simulink model "threephasedcac"  (R2016a)
settings: Solver=VariableStepAuto  StartTime=0.0  StopTime=60e-3  RelTol=1e-3
libraries: powerlib x15, powerlib_meascontrol x4
settings Model: Creator=VARUN SINGH  LastModifiedBy=VARUN SINGH

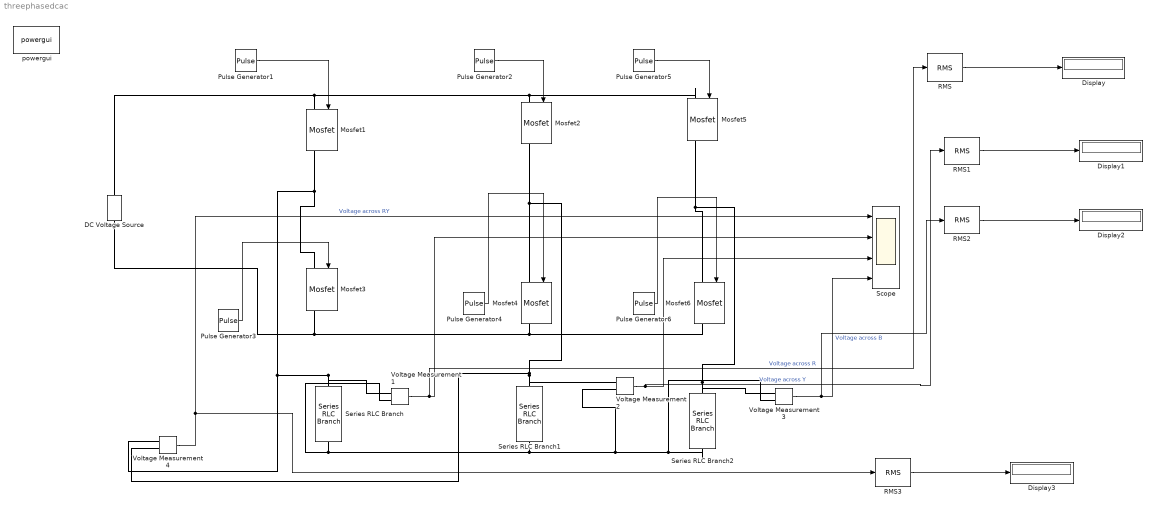
== system threephasedcac ==
  DC Voltage Source : powerlib/Electrical Sources/DC Voltage Source  Amplitude=325  Measurements=None
  Display{,1..3} (4 alike) : Display
  Mosfet{1..6} (6 alike) : powerlib/Power Electronics/Mosfet  Ron=0.1  Lon=0  Rd=0.01  Vfd=0  IC=0  Rs=1e5  Cs=inf  Measurements=on
  Pulse Generator1 : DiscretePulseGenerator  PulseType=Time based  Period=20e-3  PulseWidth=100/3
  Pulse Generator2 : DiscretePulseGenerator  PulseType=Time based  Period=20e-3  PulseWidth=100/3  PhaseDelay=(180/180)*10e-3
  Pulse Generator3 : DiscretePulseGenerator  PulseType=Time based  Period=20e-3  PulseWidth=100/3  PhaseDelay=10e-3
  Pulse Generator4 : DiscretePulseGenerator  PulseType=Time based  Period=20e-3  PulseWidth=100/3  PhaseDelay=(180/180)*10e-3+10e-3
  Pulse Generator5 : DiscretePulseGenerator  PulseType=Time based  Period=20e-3  PulseWidth=100/3  PhaseDelay=(360/180)*10e-3
  Pulse Generator6 : DiscretePulseGenerator  PulseType=Time based  Period=20e-3  PulseWidth=100/3  PhaseDelay=(360/180)*10e-3+10e-3
  RMS{,1..3} (4 alike) : powerlib_meascontrol/Measurements/RMS  TrueRMS=on  Freq=60  RMSInit=120  Ts=0
  Scope : Scope  NumInputPorts=4
  Series RLC Branch : powerlib/Elements/Series RLC Branch  LConnTagsString=__new0  RConnTagsString=__new0  BranchType=R  Resistance=100  Inductance=10e-3  SetiL0=off  InitialCurrent=0  Capacitance=1e-6  Setx0=off  InitialVoltage=0  Measurements=None
  Series RLC Branch1 : powerlib/Elements/Series RLC Branch  LConnTagsString=__new0  RConnTagsString=__new0  BranchType=R  Resistance=100  Inductance=10e-3  SetiL0=off  InitialCurrent=0  Capacitance=1e-6  Setx0=off  InitialVoltage=0  Measurements=None
  Series RLC Branch2 : powerlib/Elements/Series RLC Branch  LConnTagsString=__new0  RConnTagsString=__new0  BranchType=R  Resistance=100  Inductance=10e-3  SetiL0=off  InitialCurrent=0  Capacitance=1e-6  Setx0=off  InitialVoltage=0  Measurements=None
  Voltage Measurement{1..4} (4 alike) : powerlib/Measurements/Voltage Measurement  PhasorSimulation=off  OutputType=Complex  PSBequivalent=0
  powergui : powerlib/powergui  Priority=1  SimulationMode=Continuous  SolverType=Tustin/Backward Euler (TBE)  SampleTime=50e-6  frequency=60  SPID=off  DisableSnubberDevices=off  DisableRonSwitches=off  DisableVfSwitches=off  SwTol=0  DisplayEquations=off  Interpol=off  ExternalGateDelay=off  methode=off  Ts=10  FunctionMessages=off  echomessages=off  HookPort=off  EnableUseOfTLC=off  x0status=blocks  frequencyindice=0  Pbase=100e6  ErrMax=1e-4  Iterations=50  UnitsV=kV  UnitsW=MW  buscounter=0  RestoreLinks=warning  ResistiveCurrentMeasurement=off  Frange=[0:2:500]  Ylog=off  Xlog=on  ShowGrid=off  save=off  variable=ZData  structure=0  ZoomFFT=off  StartTime=0.0  cycles=1  DisplayStyle=1  fundamental=60  FreqAxis=off  MaxFrequency=1000  frequencyindicesteady=1  RmsSteady=1  display=off
  wires:
  Pulse Generator5/1 -> Mosfet5/1
  Pulse Generator6/1 -> Mosfet6/1
  Pulse Generator2/1 -> Mosfet2/1
  Pulse Generator4/1 -> Mosfet4/1
  Pulse Generator1/1 -> Mosfet1/1
  Pulse Generator3/1 -> Mosfet3/1
  Voltage Measurement4/1 -> RMS3/1, Scope/1  "Voltage across RY"
  Voltage Measurement1/1 -> RMS/1, Scope/2  "Voltage across R"
  Voltage Measurement2/1 -> RMS1/1, Scope/3  "Voltage across Y"
  Voltage Measurement3/1 -> RMS2/1, Scope/4  "Voltage across B"
  RMS/1 -> Display/1
  RMS2/1 -> Display2/1
  RMS1/1 -> Display1/1
  RMS3/1 -> Display3/1
  connections:
  Mosfet2/RConn1 -- Voltage Measurement4/LConn2 -- Voltage Measurement2/LConn1 -- Series RLC Branch1/RConn1 -- Mosfet4/LConn1
  Mosfet3/LConn1 -- Voltage Measurement1/LConn1 -- Series RLC Branch/RConn1 -- Voltage Measurement4/LConn1 -- Mosfet1/RConn1
  Mosfet1/LConn1 -- Mosfet5/LConn1 -- Mosfet2/LConn1 -- DC Voltage Source/RConn1
  Mosfet3/RConn1 -- Mosfet6/RConn1 -- Mosfet4/RConn1 -- DC Voltage Source/LConn1
  Mosfet5/RConn1 -- Voltage Measurement3/LConn1 -- Series RLC Branch2/RConn1 -- Mosfet6/LConn1
  Series RLC Branch/LConn1 -- Voltage Measurement3/LConn2 -- Series RLC Branch2/LConn1 -- Voltage Measurement2/LConn2 -- Series RLC Branch1/LConn1 -- Voltage Measurement1/LConn2
